simulink model "Ej_1_1"  (R2022b)
settings: Solver=VariableStepAuto  StartTime=0.0  StopTime=5  RelTol=1e-3
settings Model: Creator=rrilo  LastModifiedBy=rrilo

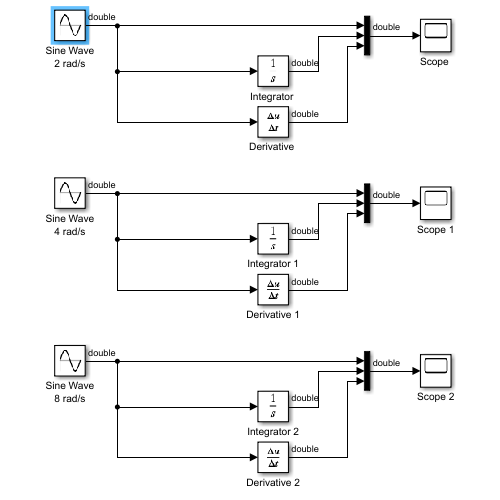
[thumbnail: Simulink's stored preview of the top-level diagram]
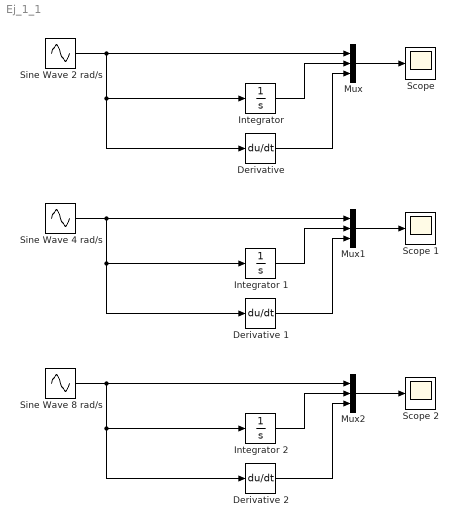
== system Ej_1_1 ==
  "Derivative " : Derivative
  Derivative 1 : Derivative
  Derivative 2 : Derivative
  "Integrator " : Integrator
  Integrator 1 : Integrator
  Integrator 2 : Integrator
  Mux : Mux  Inputs=3
  Mux1 : Mux  Inputs=3
  Mux2 : Mux  Inputs=3
  "Scope " : Scope
  Scope 1 : Scope
  Scope 2 : Scope
  Sine Wave 2 rad/s : Sin  Amplitude=2  Frequency=2  SampleTime=0
  Sine Wave 4 rad/s : Sin  Amplitude=2  Frequency=4  SampleTime=0
  Sine Wave 8 rad/s : Sin  Amplitude=2  Frequency=8  SampleTime=0
  wires:
  Sine Wave 2 rad/s/1 -> "Integrator "/1, "Derivative "/1, Mux/1
  "Integrator "/1 -> Mux/2
  "Derivative "/1 -> Mux/3
  Mux/1 -> "Scope "/1
  Sine Wave 4 rad/s/1 -> Integrator 1/1, Derivative 1/1, Mux1/1
  Derivative 1/1 -> Mux1/3
  Integrator 1/1 -> Mux1/2
  Mux1/1 -> Scope 1/1
  Sine Wave 8 rad/s/1 -> Integrator 2/1, Derivative 2/1, Mux2/1
  Derivative 2/1 -> Mux2/3
  Integrator 2/1 -> Mux2/2
  Mux2/1 -> Scope 2/1
